simulink model "sm_tVtest_roller_elem"  (R2026a)
settings: Solver=VariableStepAuto  AbsTol=1e-3  EnableMultiTasking=on
undefined symbols (not defined in the file): Excv, X, Y, Z
libraries: sm_trackV_lib_chain_underc_elem x13, sm_lib x6, sm_trackV_lib_chain_segment x3, sm_trackV_lib_frame_i1u2l7 x1, nesl_utility x1
Description:
  | Excavator Track Check Assembly Sprocket, Roller, and Idler
  | Copyright 2023-2026 The MathWorks, Inc.
settings Model: Creator=smiller  LastModifiedBy=smiller
settings DebuggingCC: SubsystemReferenceDiagnosticForUnitTest=warning
settings SimscapeCC: SimscapeNominalValues="[{\"value\":\"1\",\"unit\":\"A\"},{\"value\":\"1\",\"unit\":\"bar\"},{\"value\":\"1\",\"unit\":\"cm^2\"},{\"value\":\"1\",\"unit\":\"cm^3/s\"},{\"value\":\"1\",\"unit\":\"kJ/kg\"},{\"value\":\"1\",\"unit\":\"kW\"},{\"value\":\"1\",\"unit\":\"l\"},{\"value\":\"1\",\"unit\":\"N\"},{\"value\":\"1\",\"unit\":\"N*m\"},{\"value\":\"1\",\"unit\":\"V\"}]"  SimscapeLogSimulationStatistics=on
settings DiagnosticsConfigSet: SimMechanicsUnconnectedFramePorts=none
settings ExplorerConfigSet: InternalSimMechanicsExplorerSettings="<ExplorerConfiguration><canonicalview>default</canonicalview><AnimationSetting><BasePlaybackSpeed>1.0</BasePlaybackSpeed><PlaybackSpeedFactor>1.0</PlaybackSpeedFactor></AnimationSetting><TilePanel><TileInfo><Tiles Columns=\"1\" Count=\"1\" Rows=\"1\"><Column Weight=\"1\"/><Row Weight=\"1\"/><Tile Height=\"1\" Width=\"1\" X=\"0\" Y=\"0\"/></Tiles></TileInfo><SceneInfo><SceneViewer><BGColor><R>1</R><G>1</G><B>1</B></BGColor><Camera><DoPerspective>off</DoPerspective><Position><X>1.66029473295456342</X><Y>-0.0187233019380660948</Y><Z>2.27625898993924514</Z></Position><Center><X>1.66029473295456342</X><Y>-0.0187233019380660948</Y><Z>-1.55881308749883374e-07</Z></Center><Up><X>0</X><Y>1</Y><Z>-0</Z></Up><ViewLimDist>1</ViewLimDist><YLim>1.35491257339365334</YLim><XLim>2.0750913286209105</XLim></Camera></SceneViewer></SceneInfo></TilePanel><MechEditorPanel><Cameras/><GfxPanelCameraMap/><VideoCreator><PlaybackSpeedRatio>1.0</PlaybackSpeedRatio><FrameRate>30</FrameRate><VideoFormat>Motion JPEG AVI</VideoFormat><FrameSize>auto</FrameSize></VideoCreator></MechEditorPanel></ExplorerConfiguration>"

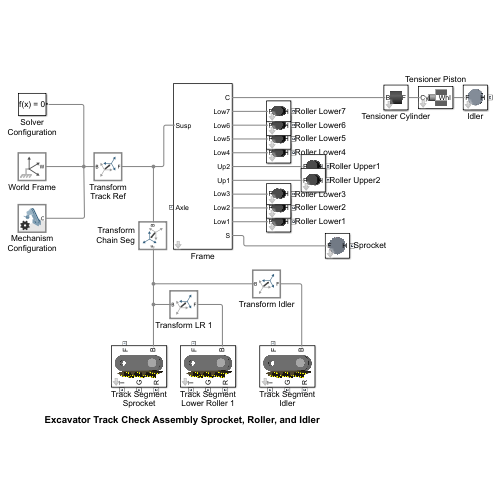
[thumbnail: Simulink's stored preview of the top-level diagram]
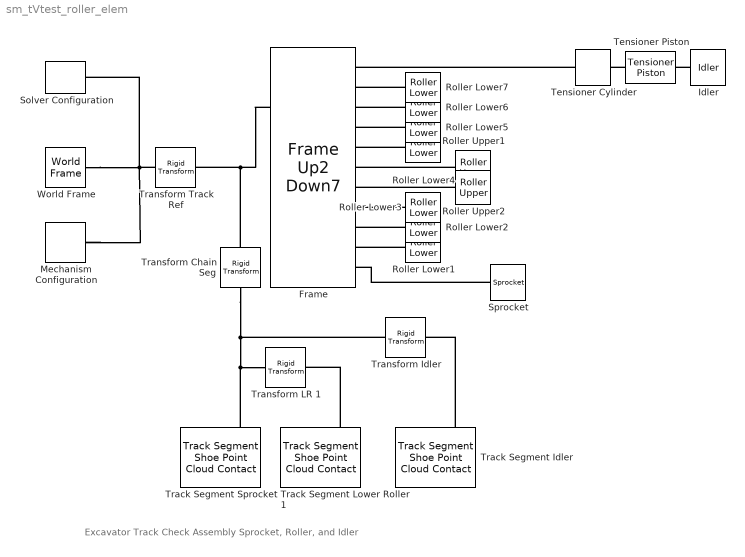
== system sm_tVtest_roller_elem ==
  note: Excavator Track Check Assembly Sprocket, Roller, and Idler
  Frame : sm_trackV_lib_frame_i1u2l7/Frame Up2 Down7  popup_leftOrRight=Right  roller_upper_x=Excv.Frame.Sprk2UpperX  roller_lower_x=Excv.Frame.Sprk2LowerX  idler_x=Excv.Frame.IdlerAssyX  axle_x=Excv.Frame.AxleX  roller_upper_y=Excv.Frame.Sprk2UpperY  roller_lower_y=Excv.Frame.Sprk2LowerY  idler_y=Excv.Frame.Sprk2IdlerY  axle_y=Excv.Frame.AxleY  frame_cg_offset=Excv.Frame.CGOffset  frame_mass=Excv.Frame.Mass  frame_moi=Excv.Frame.MOI  frame_poi=Excv.Frame.POI  frame_susp_offset=Excv.Frame.SuspOffset
  Idler : sm_trackV_lib_chain_underc_elem/Idler  idler_rad=Excv.Idler.rad  idler_len=Excv.Idler.len  idler_rho=Excv.Idler.rho  idler_clr=Excv.Idler.clr  idler_opc=Excv.Idler.opc  idler_contgeo_clr=[1.0 0.0 0.0]  idler_contgeo_opc=0
  Mechanism Configuration : sm_lib/Utilities/Mechanism Configuration  UniformGravity=Constant  GravityVector=[0 0 -9.80665]  GravityVectorUnits=m/s^2  LinearizationDelta=0.001  JointModeTransitionNonlinearIterations=2
  Roller Lower{1..7} (7 alike) : sm_trackV_lib_chain_underc_elem/Roller Lower  roller_lower_rad=Excv.Roller.Lower.rad  roller_lower_len=Excv.Roller.Lower.len  roller_lower_rho=Excv.Roller.Lower.rho  roller_lower_clr=Excv.Roller.Lower.clr  roller_lower_opc=Excv.Roller.Lower.opc  roller_lower_contgeo_clr=[1.0 0.0 0.0]  roller_lower_contgeo_opc=1
  Roller Upper1 : sm_trackV_lib_chain_underc_elem/Roller Upper  roller_upper_rad=Excv.Roller.Upper.rad  roller_upper_len=Excv.Roller.Upper.len  roller_upper_rho=Excv.Roller.Upper.rho  roller_upper_clr=Excv.Roller.Upper.clr  roller_upper_opc=Excv.Roller.Upper.opc  roller_upper_contgeo_clr=[1.0 0.0 0.0]  roller_upper_contgeo_opc=1
  Roller Upper2 : sm_trackV_lib_chain_underc_elem/Roller Upper  roller_upper_rad=Excv.Roller.Upper.rad  roller_upper_len=Excv.Roller.Upper.len  roller_upper_rho=Excv.Roller.Upper.rho  roller_upper_clr=Excv.Roller.Upper.clr  roller_upper_opc=Excv.Roller.Upper.opc  roller_upper_contgeo_clr=[1.0 0.0 0.0]  roller_upper_contgeo_opc=1
  Solver Configuration : nesl_utility/Solver Configuration  PhysicalDomain=network_engine_domain  SubClassName=solver  LeftPortType=input  RightPortType=generic  Tones=[]  Harmonics=[]  SimulateNoise=off  Profile=off  UseLocalSampling=off  EnableSwitchedLinearOptims=on  FrequencyDomain=off  UseCCode=off  RelTol=0.001  AbsTol=1e-06  MinStep=1e-09  ToWorkspace=off  RevertToSquareIcSolve=off  NumHomotopyIterations=100  PhasorMode=off  PhasorModeNumHarmonics=1  ConsistencySolver=NEWTON_XTOL_AFTER_FTOL  CanonicalOrdering=UNORDERED  OptimizeIntermediates=UNOPTIMIZED  IndexReductionMethod=DerivativeReplacement  DoDC=off  ResidualTolerance=1e-09  ConsistencyTolSource=GLOBAL  ConsistencyAbsTol=0.001  ConsistencyRelTol=0.001  ConsistencyTolFactor=0.001  UseLocalSolver=off  LocalSolverChoice=NE_BACKWARD_EULER_ADVANCER  ResolveIndetEquations=on  FunctionEvalNumThread=1  LocalSolverSampleTime=0.001  DoFixedCost=off  MaxNonlinIter=3  MaxModeIter=2  ComputeImpulses=off  ImpulseIterations=2  LinearAlgebra=Sparse  LinearAlgebraNumThread=0  EquationFormulation=NE_TIME_EF  DelaysMemoryBudget=1024  AutomaticFiltering=on  FilteringTimeConstant=0.001  PartitionStorageMethod=AS_NEEDED  PartitionMemoryBudget=1024  PartitionMethod=FAST  MultibodyUseLocalSolver=off  MultibodyLocalSolverChoice=ODE1  MultibodyLocalSolverSampleTime=0.001
  Sprocket : sm_trackV_lib_chain_underc_elem/Sprocket  sprk_xc=Excv.Sprocket.sprocket_xc  sprk_len=Excv.Sprocket.sprk_width  sprk_rho=Excv.Sprocket.density  sprk_clr=Excv.Sprocket.clr  sprk_opc=Excv.Sprocket.opc  sprk_contact_geo_ptcld=Excv.Sprocket.teeth_contact.ptcld.pts  sprk_contact_geo_rad=Excv.Sprocket.teeth_contact.ptcld.rad  sprk_contact_geo_clr=Excv.Sprocket.teeth_contact.ptcld.clr  sprk_contact_geo_opc=Excv.Sprocket.teeth_contact.ptcld.opc
  Tensioner Cylinder : sm_trackV_lib_chain_underc_elem/Tensioner Cylinder  cyl_rad=Excv.Idler.Tensioner.cyl.rad  cyl_len=Excv.Idler.Tensioner.cyl.len  cyl_rho=Excv.Idler.Tensioner.cyl.rho  cyl_clr=Excv.Idler.Tensioner.cyl.clr  cyl_opc=Excv.Idler.Tensioner.cyl.opc  brk_len=Excv.Idler.Tensioner.bracket.len  brk_thk=Excv.Idler.Tensioner.bracket.thk  pist_len=Excv.Idler.Tensioner.piston.len
  Tensioner Piston : sm_trackV_lib_chain_underc_elem/Tensioner Piston  pist_rad=Excv.Idler.Tensioner.piston.rad  pist_len=Excv.Idler.Tensioner.piston.len  pist_rho=Excv.Idler.Tensioner.piston.rho  pist_clr=Excv.Idler.Tensioner.piston.clr  pist_opc=Excv.Idler.Tensioner.piston.opc  br_height=Excv.Idler.Tensioner.bracket.height  br_length=Excv.Idler.Tensioner.bracket.len  br_width=Excv.Idler.Tensioner.bracket.wid  br_rho=Excv.Idler.Tensioner.bracket.rho  br_thk=Excv.Idler.Tensioner.bracket.thk  br_clr=Excv.Idler.Tensioner.bracket.clr  br_opc=Excv.Idler.Tensioner.bracket.opc
  Track Segment Idler : sm_trackV_lib_chain_segment/Track Segment Shoe Point Cloud Contact  chain_wid=Excv.Chain.chain_wid  chain_seg_m=Excv.Chain.link_m  chain_seg_cg=Excv.Chain.link_cg  chain_seg_moi=Excv.Chain.link_moi  chain_seg_poi=Excv.Chain.link_poi  plate_h=Excv.Chain.plate_h  plate_xc=Excv.Chain.plate_xc  plate_thk=Excv.Chain.plate_thk  pin_sep=Excv.Chain.pin_sep  plate_ang=Excv.Chain.plate_ang  plate_clr=Excv.Chain.plate_clr  plate_opc=1  pin_len=Excv.Chain.pin_len  pin_rad=Excv.Chain.pin_rad  pin_clr=Excv.Chain.pin_clr  pin_opc=1  shoe_xc=Excv.Shoe.xc  shoe_w=Excv.Shoe.w  shoe_m=Excv.Shoe.mass  shoe_cg=Excv.Shoe.cg  shoe_moi=Excv.Shoe.moi  shoe_poi=Excv.Shoe.poi  shoe_clr=Excv.Shoe.clr  shoe_opc=1  posTgtSpecify=on  posTgtPriority=High  PositionTargetValue=0  DampingCoefficient=1.0  ptcld_shoe=Excv.Shoe.ground_contact.ptcld.pts  ptcld_shoe_rad=Excv.Shoe.ground_contact.ptcld.rad  ptcld_shoe_clr=Excv.Shoe.ground_contact.ptcld.clr  ptcld_shoe_opc=Excv.Shoe.ground_contact.ptcld.opc  chain_to_roller_clr=[1.0 0.0 0.2]  chain_to_roller_opc=0.5  chain_to_teeth_clr=[1.0 0.0 0.0]  chain_to_teeth_opc=0.5
  Track Segment Lower Roller 1 : sm_trackV_lib_chain_segment/Track Segment Shoe Point Cloud Contact  chain_wid=Excv.Chain.chain_wid  chain_seg_m=Excv.Chain.link_m  chain_seg_cg=Excv.Chain.link_cg  chain_seg_moi=Excv.Chain.link_moi  chain_seg_poi=Excv.Chain.link_poi  plate_h=Excv.Chain.plate_h  plate_xc=Excv.Chain.plate_xc  plate_thk=Excv.Chain.plate_thk  pin_sep=Excv.Chain.pin_sep  plate_ang=Excv.Chain.plate_ang  plate_clr=Excv.Chain.plate_clr  plate_opc=1  pin_len=Excv.Chain.pin_len  pin_rad=Excv.Chain.pin_rad  pin_clr=Excv.Chain.pin_clr  pin_opc=1  shoe_xc=Excv.Shoe.xc  shoe_w=Excv.Shoe.w  shoe_m=Excv.Shoe.mass  shoe_cg=Excv.Shoe.cg  shoe_moi=Excv.Shoe.moi  shoe_poi=Excv.Shoe.poi  shoe_clr=Excv.Shoe.clr  shoe_opc=1  posTgtSpecify=on  posTgtPriority=High  PositionTargetValue=0  DampingCoefficient=1.0  ptcld_shoe=Excv.Shoe.ground_contact.ptcld.pts  ptcld_shoe_rad=Excv.Shoe.ground_contact.ptcld.rad  ptcld_shoe_clr=Excv.Shoe.ground_contact.ptcld.clr  ptcld_shoe_opc=Excv.Shoe.ground_contact.ptcld.opc  chain_to_roller_clr=[1.0 0.0 0.2]  chain_to_roller_opc=0.5  chain_to_teeth_clr=[1.0 0.0 0.0]  chain_to_teeth_opc=0.5
  Track Segment Sprocket : sm_trackV_lib_chain_segment/Track Segment Shoe Point Cloud Contact  chain_wid=Excv.Chain.chain_wid  chain_seg_m=Excv.Chain.link_m  chain_seg_cg=Excv.Chain.link_cg  chain_seg_moi=Excv.Chain.link_moi  chain_seg_poi=Excv.Chain.link_poi  plate_h=Excv.Chain.plate_h  plate_xc=Excv.Chain.plate_xc  plate_thk=Excv.Chain.plate_thk  pin_sep=Excv.Chain.pin_sep  plate_ang=Excv.Chain.plate_ang  plate_clr=Excv.Chain.plate_clr  plate_opc=1  pin_len=Excv.Chain.pin_len  pin_rad=Excv.Chain.pin_rad  pin_clr=Excv.Chain.pin_clr  pin_opc=1  shoe_xc=Excv.Shoe.xc  shoe_w=Excv.Shoe.w  shoe_m=Excv.Shoe.mass  shoe_cg=Excv.Shoe.cg  shoe_moi=Excv.Shoe.moi  shoe_poi=Excv.Shoe.poi  shoe_clr=Excv.Shoe.clr  shoe_opc=1  posTgtSpecify=on  posTgtPriority=High  PositionTargetValue=0  DampingCoefficient=1.0  ptcld_shoe=Excv.Shoe.ground_contact.ptcld.pts  ptcld_shoe_rad=Excv.Shoe.ground_contact.ptcld.rad  ptcld_shoe_clr=Excv.Shoe.ground_contact.ptcld.clr  ptcld_shoe_opc=Excv.Shoe.ground_contact.ptcld.opc  chain_to_roller_clr=[1.0 0.0 0.2]  chain_to_roller_opc=0.5  chain_to_teeth_clr=[1.0 0.0 0.0]  chain_to_teeth_opc=0.5
  Transform Chain Seg : sm_lib/Frames and Transforms/Rigid Transform  RotationMethod=StandardAxis  FollAlignAxisA=+X  BaseAlignAxisA=+Y  FollAlignAxisB=+Y  BaseAlignAxisB=+Z  RotationStandardAxis=+Z  RotationAngle=180  RotationAngleUnits=deg  RotationArbitraryAxis=[0 0 1]  RotationSequenceAxes=FollowerAxes  RotationSequence=XYX  RotationSequenceAngles=[0 0 0]  RotationSequenceAnglesUnits=deg  RotationMatrix=[1 0 0; 0 1 0; 0 0 1]  Quaternion=[1 0 0 0]  TranslationMethod=StandardAxis  TranslationCartesianOffset=[0 0 0]  TranslationCartesianOffsetUnits=m  TranslationStandardAxis=+Y  TranslationStandardOffset=Excv.Sprocket.sprocket_rPitch  TranslationStandardOffsetUnits=m  TranslationROffset=0  TranslationROffsetUnits=m  TranslationThetaOffset=0  TranslationThetaOffsetUnits=deg  TranslationZOffset=0  TranslationZOffsetUnits=m
  Transform Track Ref : sm_lib/Frames and Transforms/Rigid Transform  RotationMethod=StandardAxis  FollAlignAxisA=+X  BaseAlignAxisA=+Y  FollAlignAxisB=+Y  BaseAlignAxisB=+Z  RotationStandardAxis=+X  RotationAngle=180  RotationAngleUnits=deg  RotationArbitraryAxis=[0 0 1]  RotationSequenceAxes=FollowerAxes  RotationSequence=XYX  RotationSequenceAngles=[0 0 0]  RotationSequenceAnglesUnits=deg  RotationMatrix=[1 0 0; 0 1 0; 0 0 1]  Quaternion=[1 0 0 0]  TranslationMethod=None  TranslationCartesianOffset=[0 0 0]  TranslationCartesianOffsetUnits=m  TranslationStandardAxis=+Z  TranslationStandardOffset=0  TranslationStandardOffsetUnits=m  TranslationROffset=0  TranslationROffsetUnits=m  TranslationThetaOffset=0  TranslationThetaOffsetUnits=deg  TranslationZOffset=0  TranslationZOffsetUnits=m
  Transform Idler : sm_lib/Frames and Transforms/Rigid Transform  RotationMethod=None  FollAlignAxisA=+X  BaseAlignAxisA=+Y  FollAlignAxisB=+Y  BaseAlignAxisB=+Z  RotationStandardAxis=+X  RotationAngle=180  RotationAngleUnits=deg  RotationArbitraryAxis=[0 0 1]  RotationSequenceAxes=FollowerAxes  RotationSequence=XYX  RotationSequenceAngles=[0 0 0]  RotationSequenceAnglesUnits=deg  RotationMatrix=[1 0 0; 0 1 0; 0 0 1]  Quaternion=[1 0 0 0]  TranslationMethod=StandardAxis  TranslationCartesianOffset=[0 0 0]  TranslationCartesianOffsetUnits=m  TranslationStandardAxis=+X  TranslationStandardOffset=-Excv.Frame.IdlerAssyX+Excv.Chain.pin_sep/2  TranslationStandardOffsetUnits=m  TranslationROffset=0  TranslationROffsetUnits=m  TranslationThetaOffset=0  TranslationThetaOffsetUnits=deg  TranslationZOffset=0  TranslationZOffsetUnits=m
  Transform LR 1 : sm_lib/Frames and Transforms/Rigid Transform  RotationMethod=None  FollAlignAxisA=+X  BaseAlignAxisA=+Y  FollAlignAxisB=+Y  BaseAlignAxisB=+Z  RotationStandardAxis=+X  RotationAngle=180  RotationAngleUnits=deg  RotationArbitraryAxis=[0 0 1]  RotationSequenceAxes=FollowerAxes  RotationSequence=XYX  RotationSequenceAngles=[0 0 0]  RotationSequenceAnglesUnits=deg  RotationMatrix=[1 0 0; 0 1 0; 0 0 1]  Quaternion=[1 0 0 0]  TranslationMethod=StandardAxis  TranslationCartesianOffset=[0 0 0]  TranslationCartesianOffsetUnits=m  TranslationStandardAxis=+X  TranslationStandardOffset=-(Excv.Frame.Sprk2LowerX(1)-Excv.Chain.pin_sep/2)  TranslationStandardOffsetUnits=m  TranslationROffset=0  TranslationROffsetUnits=m  TranslationThetaOffset=0  TranslationThetaOffsetUnits=deg  TranslationZOffset=0  TranslationZOffsetUnits=m
  World Frame : sm_lib/Frames and Transforms/World Frame
  connections:
  Frame/LConn1 -- Transform Track Ref/RConn1 -- Transform Chain Seg/LConn1
  Roller Lower1/LConn1 -- Frame/RConn10
  Roller Lower6/LConn1 -- Frame/RConn3
  Roller Lower5/LConn1 -- Frame/RConn4
  Roller Lower4/LConn1 -- Frame/RConn5
  Roller Upper1/LConn1 -- Frame/RConn6
  Roller Upper2/LConn1 -- Frame/RConn7
  Roller Lower3/LConn1 -- Frame/RConn8
  Roller Lower2/LConn1 -- Frame/RConn9
  Tensioner Cylinder/LConn1 -- Frame/RConn1
  Roller Lower7/LConn1 -- Frame/RConn2
  Sprocket/LConn1 -- Frame/RConn11
  Tensioner Piston/LConn1 -- Tensioner Cylinder/RConn1
  Idler/LConn1 -- Tensioner Piston/RConn1
  Transform Track Ref/LConn1 -- Mechanism Configuration/RConn1 -- World Frame/RConn1 -- Solver Configuration/RConn1
  Transform Chain Seg/RConn1 -- Transform Idler/LConn1 -- Track Segment Sprocket/LConn1 -- Transform LR 1/LConn1
  Track Segment Lower Roller 1/LConn1 -- Transform LR 1/RConn1
  Track Segment Idler/LConn1 -- Transform Idler/RConn1
